simulink model "motion_detection"  (Simulink 7.3)
settings: Solver=ode45  StartTime=0.0  StopTime=15  RelTol=1e-3
undefined symbols (not defined in the file): Rec, SDTV, ttNCM
libraries: truetime x9, dspsigops x6, vipconversions x4, vipanalysis x4, vipgeotforms x4, dspobslib x4, dspsrcs4 x4, vipsnks x1
settings Model: Creator=Ayush Gupta  LastModifiedBy=Ayush Gupta
settings SimEventsCC: propDiagAttribOutput=1  propDiagFcnCallOutput=1  propDiagStatOutput=0

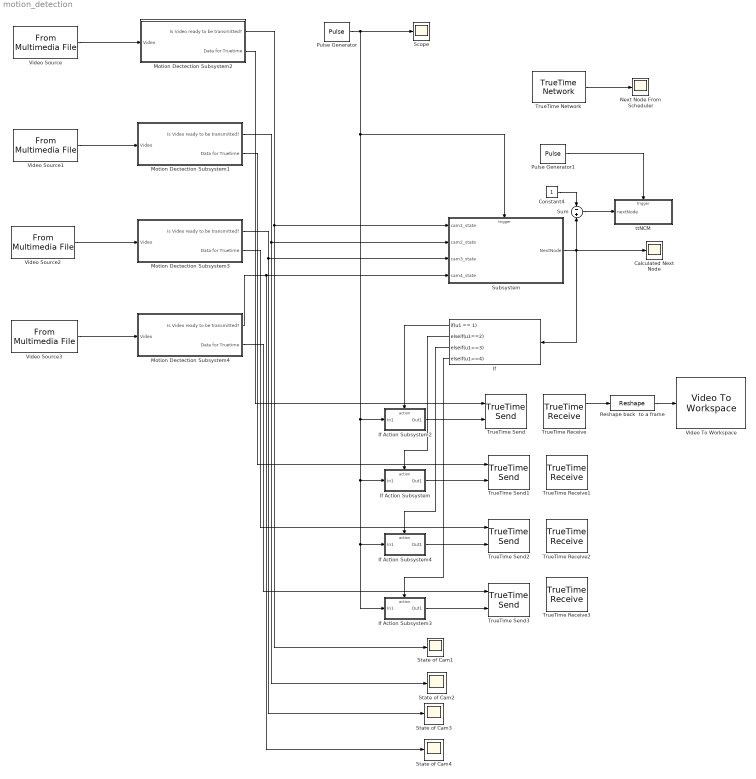
== system motion_detection ==
  Calculated Next Node : Scope
      settings: YMin=0  YMax=4
  Constant4 : Constant  OutDataType=fixdt(1, 16)  OutScaling=2^0
  If : If  IfExpression=u1 == 1  ElseIfExpressions=u1==2,u1==3,u1==4  ShowElse=off
  If Action Subsystem : Subsystem  TreatAsAtomicUnit=on
  If Action Subsystem2 : Subsystem  TreatAsAtomicUnit=on
  If Action Subsystem3 : Subsystem  TreatAsAtomicUnit=on
  If Action Subsystem4 : Subsystem  TreatAsAtomicUnit=on
  Motion Dectection Subsystem1 : Subsystem
  Motion Dectection Subsystem2 : Subsystem
  Motion Dectection Subsystem3 : Subsystem
  Motion Dectection Subsystem4 : Subsystem
  Next Node From Scheduler : Scope
      settings: YMin=1  YMax=4.5  SaveName=ScopeData5
  Pulse Generator : DiscretePulseGenerator  PulseType=Time based  Amplitude=1  Period=0.1  PulseWidth=10  PhaseDelay=0  SampleTime=1
  Pulse Generator1 : DiscretePulseGenerator  PulseType=Time based  Amplitude=1  Period=0.05  PulseWidth=10  PhaseDelay=0  SampleTime=1
  Reshape back  to a frame : Reshape  OutputDimensionality=Customize  OutputDimensions=[120,160,3]
  Scope : Scope
      settings: YMin=-1  YMax=1
  State of Cam{1..4} (4 alike) : Scope
      State of Cam1 settings: YMin=0  YMax=4  SaveName=ScopeData2
      State of Cam2 settings: YMin=0  YMax=4  SaveName=ScopeData3
      State of Cam3 settings: YMin=0  YMax=4  SaveName=ScopeData4
      State of Cam4 settings: YMin=0  YMax=4  SaveName=ScopeData6
  Subsystem : Subsystem
      settings: MinAlgLoopOccurrences=on
  Sum : Sum  Inputs=-+  OutDataType=sfix(16)  OutScaling=2^0  OutDataTypeStr=Inherit: Same as first input
  TrueTime Network : truetime/TrueTime Network  SystemSampleTime=-1  nwtype=NCM  nwnbr=1  nnodes=4  rate=10000  minsize=512  lossprob=0  seed=0  bandwidths=[0.5 0.5]  slotsize=512  schedule=[1 1 2]  memsize=80000  buftype=Common buffer  overflow=Retransmit  dynSchedule=0  miniSlotSize=0  NIT=0  QSortMode=FIFO  sync=0  irtSchedule=0  nrtLength=0  nodeGraph=0  scheduleoutput=on
  TrueTime Receive : truetime/TrueTime Receive  SystemSampleTime=-1  nwnbr=1  receiver=1  outdim=57600  triggeroutput=on  senderoutput=off  lengthoutput=off  priorityoutput=off  timestampoutput=off  signalpoweroutput=off  msgIDoutput=off
  TrueTime Receive1 : truetime/TrueTime Receive  SystemSampleTime=-1  nwnbr=1  receiver=2  outdim=57600  triggeroutput=on  senderoutput=off  lengthoutput=off  priorityoutput=off  timestampoutput=off  signalpoweroutput=off  msgIDoutput=off
  TrueTime Receive2 : truetime/TrueTime Receive  SystemSampleTime=-1  nwnbr=1  receiver=3  outdim=57600  triggeroutput=on  senderoutput=off  lengthoutput=off  priorityoutput=off  timestampoutput=off  signalpoweroutput=off  msgIDoutput=off
  TrueTime Receive3 : truetime/TrueTime Receive  SystemSampleTime=-1  nwnbr=1  receiver=4  outdim=57600  triggeroutput=on  senderoutput=off  lengthoutput=off  priorityoutput=off  timestampoutput=off  signalpoweroutput=off  msgIDoutput=off
  TrueTime Send : truetime/TrueTime Send  SystemSampleTime=-1  trigger=falling  nwnbr=1  sender=1  indim=57600  recsource=internal  receiver=1  lengthsource=internal  length=1000  priosource=internal  prio=1  msgIDsource=internal  msgID=0  dynamicSegment=dynamic
  TrueTime Send1 : truetime/TrueTime Send  SystemSampleTime=-1  trigger=falling  nwnbr=1  sender=2  indim=57600  recsource=internal  receiver=1  lengthsource=internal  length=1000  priosource=internal  prio=1  msgIDsource=internal  msgID=0  dynamicSegment=dynamic
  TrueTime Send2 : truetime/TrueTime Send  SystemSampleTime=-1  trigger=falling  nwnbr=1  sender=3  indim=57600  recsource=internal  receiver=1  lengthsource=internal  length=1000  priosource=internal  prio=1  msgIDsource=internal  msgID=0  dynamicSegment=dynamic
  TrueTime Send3 : truetime/TrueTime Send  SystemSampleTime=-1  trigger=falling  nwnbr=1  sender=4  indim=57600  recsource=internal  receiver=1  lengthsource=internal  length=1000  priosource=internal  prio=1  msgIDsource=internal  msgID=0  dynamicSegment=dynamic
  Video Source : dspsrcs4/From Multimedia File  DialogController=dspDDGCreate  DialogControllerArgs=DataTag8  inputFilename=C:\Users\Ayush Gupta\truetime\examples\NCM\VideoModel\InputVideo\vipmen.avi  loop=on  numPlays=inf  outputStreams=Video only  videoDataType=double  audioDataType=int16  inheritSampleTime=on  userDefinedSampleTime=1/30  noAudioOutput=off  isIntensityVideo=off  colorVideoFormat=One multidimensional signal  outputEOF=off  dataOrg=Column-major  audioFrameSize=1024
  Video Source1 : dspsrcs4/From Multimedia File  DialogController=dspDDGCreate  DialogControllerArgs=DataTag9  inputFilename=C:\Users\Ayush Gupta\truetime\examples\NCM\VideoModel\InputVideo\viptraffic.avi  loop=on  numPlays=inf  outputStreams=Video only  videoDataType=double  audioDataType=int16  inheritSampleTime=on  userDefinedSampleTime=1/30  noAudioOutput=off  isIntensityVideo=off  colorVideoFormat=One multidimensional signal  outputEOF=off  dataOrg=Column-major  audioFrameSize=1024
  Video Source2 : dspsrcs4/From Multimedia File  DialogController=dspDDGCreate  DialogControllerArgs=DataTag10  inputFilename=C:\Users\Ayush Gupta\truetime\examples\NCM\VideoModel\InputVideo\Surveillance1.wmv  loop=on  numPlays=inf  outputStreams=Video only  videoDataType=double  audioDataType=int16  inheritSampleTime=on  userDefinedSampleTime=1/30  noAudioOutput=off  isIntensityVideo=off  colorVideoFormat=One multidimensional signal  outputEOF=off  dataOrg=Column-major  audioFrameSize=1024
  Video Source3 : dspsrcs4/From Multimedia File  DialogController=dspDDGCreate  DialogControllerArgs=DataTag11  inputFilename=C:\Users\Ayush Gupta\truetime\examples\NCM\VideoModel\InputVideo\Surveillance2.wmv  loop=on  numPlays=inf  outputStreams=Video only  videoDataType=double  audioDataType=int16  inheritSampleTime=on  userDefinedSampleTime=1/30  noAudioOutput=off  isIntensityVideo=off  colorVideoFormat=One multidimensional signal  outputEOF=off  dataOrg=Column-major  audioFrameSize=1024
  Video To Workspace : vipsnks/Video To Workspace  DialogController=vipDDGCreate  DialogControllerArgs=DataTag12  VariableName=TestVideo  NumInputs=1  DataLimit=inf  DecimationFactor=1  LogFi=off  InPortLabels=R|G|B
  ttNCM : Subsystem  mask(ttNCM Wrapper){nNbr=1}
      mask prompts: nNbr "networkNbr"
      mask help: Specify the Network Number
  wires:
  Video Source/1 -> Motion Dectection Subsystem2/1(Video)
  Motion Dectection Subsystem2/1(Is Video ready to be transmitted?) -> Subsystem/1(cam1_state), State of Cam1/1
  Pulse Generator/1 -> Scope/1, Subsystem/Trigger, If Action Subsystem3/1(In1), If Action Subsystem4/1(In1), If Action Subsystem/1(In1), If Action Subsystem2/1(In1)
  Subsystem/1(NextNode) -> If/1, Calculated Next Node/1, Sum/2
  If Action Subsystem2/1(Out1) -> TrueTime Send/2
  If Action Subsystem/1(Out1) -> TrueTime Send1/2
  If Action Subsystem4/1(Out1) -> TrueTime Send2/2
  If Action Subsystem3/1(Out1) -> TrueTime Send3/2
  TrueTime Network/1 -> Next Node From Scheduler/1
  Constant4/1 -> Sum/1
  Sum/1 -> ttNCM/1(nextNode)
  Pulse Generator1/1 -> ttNCM/Trigger
  TrueTime Receive/1 -> Reshape back  to a frame/1
  Reshape back  to a frame/1 -> Video To Workspace/1
  Video Source3/1 -> Motion Dectection Subsystem4/1(Video)
  Video Source2/1 -> Motion Dectection Subsystem3/1(Video)
  Video Source1/1 -> Motion Dectection Subsystem1/1(Video)
  Motion Dectection Subsystem1/1(Is Video ready to be transmitted?) -> Subsystem/2(cam2_state), State of Cam2/1
  Motion Dectection Subsystem3/1(Is Video ready to be transmitted?) -> Subsystem/3(cam3_state), State of Cam3/1
  Motion Dectection Subsystem2/2(Data for Truetime) -> TrueTime Send/1
  Motion Dectection Subsystem4/1(Is Video ready to be transmitted?) -> Subsystem/4(cam4_state), State of Cam4/1
  If/1 -> If Action Subsystem2/Action
  If/2 -> If Action Subsystem/Action
  If/3 -> If Action Subsystem4/Action
  If/4 -> If Action Subsystem3/Action
  Motion Dectection Subsystem1/2(Data for Truetime) -> TrueTime Send1/1
  Motion Dectection Subsystem3/2(Data for Truetime) -> TrueTime Send2/1
  Motion Dectection Subsystem4/2(Data for Truetime) -> TrueTime Send3/1

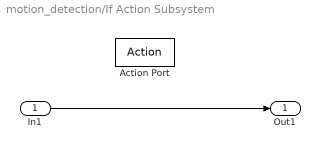
== system motion_detection/If Action Subsystem ==
  In1 : Inport  OutDataType=fixdt(1, 16)  OutScaling=2^0
  Action Port : ActionPort  ActionType=elseif
  Out1 : Outport  OutDataType=fixdt(1, 16)  OutScaling=2^0
  wires:
  In1/1 -> Out1/1

== system motion_detection/If Action Subsystem2 ==
  In1 : Inport  OutDataType=fixdt(1, 16)  OutScaling=2^0
  Action Port : ActionPort  ActionType=then
  Out1 : Outport  OutDataType=fixdt(1, 16)  OutScaling=2^0
  wires:
  In1/1 -> Out1/1

== system motion_detection/If Action Subsystem3 ==
  In1 : Inport  OutDataType=fixdt(1, 16)  OutScaling=2^0
  Action Port : ActionPort  ActionType=elseif
  Out1 : Outport  OutDataType=fixdt(1, 16)  OutScaling=2^0
  wires:
  In1/1 -> Out1/1

== system motion_detection/If Action Subsystem4 ==
  In1 : Inport  OutDataType=fixdt(1, 16)  OutScaling=2^0
  Action Port : ActionPort  ActionType=elseif
  Out1 : Outport  OutDataType=fixdt(1, 16)  OutScaling=2^0
  wires:
  In1/1 -> Out1/1

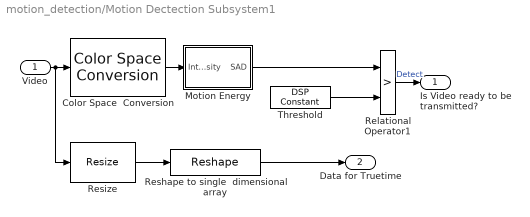
== system motion_detection/Motion Dectection Subsystem1 ==
  Video : Inport
  Color Space  Conversion : vipconversions/Color Space  Conversion  conversion=Obsolete  conversionActive=R'G'B' to intensity  wp_str=D65  rec=Rec. 601 (SDTV)  sys=1125/60/2:1  imagePorts=One multidimensional signal
  Motion Energy : Subsystem
  Relational Operator1 : RelationalOperator  Operator=>  LogicOutDataTypeMode=boolean  OutDataTypeStr=boolean  InputSameDT=on
  Reshape to single  dimensional array : Reshape
  Resize : vipgeotforms/Resize  DialogController=vipDDGCreate  DialogControllerArgs=DataTag1  specify=Number of output rows and columns  rfactor=[200 150]  outCols=25  outRows=25  outRowsCols=[120 160]  interp_method=Bilinear  antialias=on  useROI=off  roiFlag=off  prodOutputMode=Binary point scaling  prodOutputWordLength=32  prodOutputFracLength=10  roundingMode=Nearest  overflowMode=on
  Threshold : dspobslib/DSP Constant  SystemSampleTime=-1  Value=1e5/(255)  SampleMode=Discrete  discreteOutput=Sample-based  continuousOutput=Sample-based  sampTime=inf  framePeriod=inf  dataType=Inherit via back propagation  isSigned=on  wordLen=16  udDataType=sfix(16)  fracBitsMode=Best precision  numFracBits=15  InterpretAs1D=off  Ts=inf  FramebasedOutput=off
      settings: additionalParams=on
  Is Video ready to be transmitted? : Outport
  Data for Truetime : Outport  Port=2
  wires:
  Motion Energy/1(SAD) -> Relational Operator1/1
  Threshold/1 -> Relational Operator1/2
  Video/1 -> Color Space  Conversion/1, Resize/1
  Relational Operator1/1 -> Is Video ready to be transmitted?/1  "Detect"
  Color Space  Conversion/1 -> Motion Energy/1(Intensity)
  Reshape to single  dimensional array/1 -> Data for Truetime/1
  Resize/1 -> Reshape to single  dimensional array/1

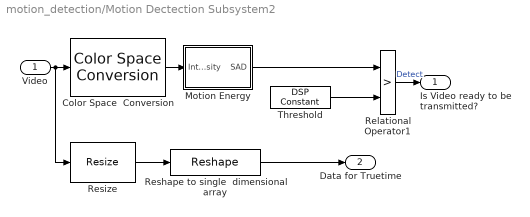
== system motion_detection/Motion Dectection Subsystem2 ==
  Video : Inport
  Color Space  Conversion : vipconversions/Color Space  Conversion  conversion=Obsolete  conversionActive=R'G'B' to intensity  wp_str=D65  rec=Rec. 601 (SDTV)  sys=1125/60/2:1  imagePorts=One multidimensional signal
  Motion Energy : Subsystem
  Relational Operator1 : RelationalOperator  Operator=>  LogicOutDataTypeMode=boolean  OutDataTypeStr=boolean  InputSameDT=on
  Reshape to single  dimensional array : Reshape
  Resize : vipgeotforms/Resize  DialogController=vipDDGCreate  DialogControllerArgs=DataTag3  specify=Number of output rows and columns  rfactor=[200 150]  outCols=25  outRows=25  outRowsCols=[120 160]  interp_method=Bilinear  antialias=on  useROI=off  roiFlag=off  prodOutputMode=Binary point scaling  prodOutputWordLength=32  prodOutputFracLength=10  roundingMode=Nearest  overflowMode=on
  Threshold : dspobslib/DSP Constant  SystemSampleTime=-1  Value=1e5/(255)  SampleMode=Discrete  discreteOutput=Sample-based  continuousOutput=Sample-based  sampTime=inf  framePeriod=inf  dataType=Inherit via back propagation  isSigned=on  wordLen=16  udDataType=sfix(16)  fracBitsMode=Best precision  numFracBits=15  InterpretAs1D=off  Ts=inf  FramebasedOutput=off
      settings: additionalParams=on
  Is Video ready to be transmitted? : Outport
  Data for Truetime : Outport  Port=2
  wires:
  Motion Energy/1(SAD) -> Relational Operator1/1
  Threshold/1 -> Relational Operator1/2
  Video/1 -> Color Space  Conversion/1, Resize/1
  Relational Operator1/1 -> Is Video ready to be transmitted?/1  "Detect"
  Color Space  Conversion/1 -> Motion Energy/1(Intensity)
  Reshape to single  dimensional array/1 -> Data for Truetime/1
  Resize/1 -> Reshape to single  dimensional array/1

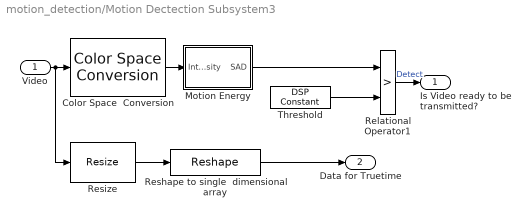
== system motion_detection/Motion Dectection Subsystem3 ==
  Video : Inport
  Color Space  Conversion : vipconversions/Color Space  Conversion  conversion=Obsolete  conversionActive=R'G'B' to intensity  wp_str=D65  rec=Rec. 601 (SDTV)  sys=1125/60/2:1  imagePorts=One multidimensional signal
  Motion Energy : Subsystem
  Relational Operator1 : RelationalOperator  Operator=>  LogicOutDataTypeMode=boolean  OutDataTypeStr=boolean  InputSameDT=on
  Reshape to single  dimensional array : Reshape
  Resize : vipgeotforms/Resize  DialogController=vipDDGCreate  DialogControllerArgs=DataTag5  specify=Number of output rows and columns  rfactor=[200 150]  outCols=25  outRows=25  outRowsCols=[120 160]  interp_method=Bilinear  antialias=on  useROI=off  roiFlag=off  prodOutputMode=Binary point scaling  prodOutputWordLength=32  prodOutputFracLength=10  roundingMode=Nearest  overflowMode=on
  Threshold : dspobslib/DSP Constant  SystemSampleTime=-1  Value=1e5/(255)  SampleMode=Discrete  discreteOutput=Sample-based  continuousOutput=Sample-based  sampTime=inf  framePeriod=inf  dataType=Inherit via back propagation  isSigned=on  wordLen=16  udDataType=sfix(16)  fracBitsMode=Best precision  numFracBits=15  InterpretAs1D=off  Ts=inf  FramebasedOutput=off
      settings: additionalParams=on
  Is Video ready to be transmitted? : Outport
  Data for Truetime : Outport  Port=2
  wires:
  Motion Energy/1(SAD) -> Relational Operator1/1
  Threshold/1 -> Relational Operator1/2
  Video/1 -> Color Space  Conversion/1, Resize/1
  Relational Operator1/1 -> Is Video ready to be transmitted?/1  "Detect"
  Color Space  Conversion/1 -> Motion Energy/1(Intensity)
  Reshape to single  dimensional array/1 -> Data for Truetime/1
  Resize/1 -> Reshape to single  dimensional array/1

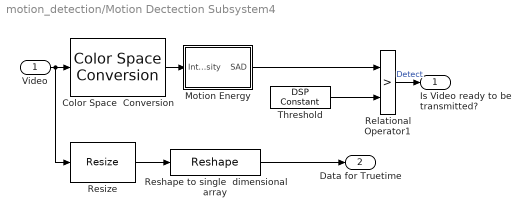
== system motion_detection/Motion Dectection Subsystem4 ==
  Video : Inport
  Color Space  Conversion : vipconversions/Color Space  Conversion  conversion=Obsolete  conversionActive=R'G'B' to intensity  wp_str=D65  rec=Rec. 601 (SDTV)  sys=1125/60/2:1  imagePorts=One multidimensional signal
  Motion Energy : Subsystem
  Relational Operator1 : RelationalOperator  Operator=>  LogicOutDataTypeMode=boolean  OutDataTypeStr=boolean  InputSameDT=on
  Reshape to single  dimensional array : Reshape
  Resize : vipgeotforms/Resize  DialogController=vipDDGCreate  DialogControllerArgs=DataTag7  specify=Number of output rows and columns  rfactor=[200 150]  outCols=25  outRows=25  outRowsCols=[120 160]  interp_method=Bilinear  antialias=on  useROI=off  roiFlag=off  prodOutputMode=Binary point scaling  prodOutputWordLength=32  prodOutputFracLength=10  roundingMode=Nearest  overflowMode=on
  Threshold : dspobslib/DSP Constant  SystemSampleTime=-1  Value=1e5/(255)  SampleMode=Discrete  discreteOutput=Sample-based  continuousOutput=Sample-based  sampTime=inf  framePeriod=inf  dataType=Inherit via back propagation  isSigned=on  wordLen=16  udDataType=sfix(16)  fracBitsMode=Best precision  numFracBits=15  InterpretAs1D=off  Ts=inf  FramebasedOutput=off
      settings: additionalParams=on
  Is Video ready to be transmitted? : Outport
  Data for Truetime : Outport  Port=2
  wires:
  Motion Energy/1(SAD) -> Relational Operator1/1
  Threshold/1 -> Relational Operator1/2
  Video/1 -> Color Space  Conversion/1, Resize/1
  Relational Operator1/1 -> Is Video ready to be transmitted?/1  "Detect"
  Color Space  Conversion/1 -> Motion Energy/1(Intensity)
  Reshape to single  dimensional array/1 -> Data for Truetime/1
  Resize/1 -> Reshape to single  dimensional array/1

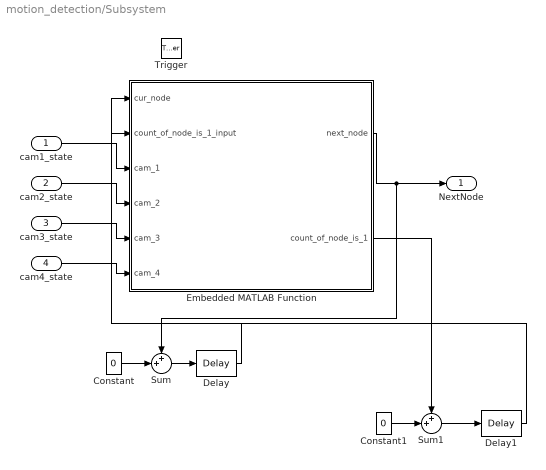
== system motion_detection/Subsystem ==
  cam1_state : Inport  OutDataType=fixdt(1, 16)  OutScaling=2^0
  cam2_state : Inport  Port=2  OutDataType=fixdt(1, 16)  OutScaling=2^0
  cam3_state : Inport  Port=3  OutDataType=fixdt(1, 16)  OutScaling=2^0
  cam4_state : Inport  Port=4  OutDataType=fixdt(1, 16)  OutScaling=2^0
  Trigger : TriggerPort  TriggerType=falling
  Constant : Constant  Value=0  OutDataTypeMode=int32  OutDataType=sfix(16)  OutScaling=2^0  OutDataTypeStr=int32
  Constant1 : Constant  Value=0  OutDataTypeMode=int32  OutDataType=sfix(16)  OutScaling=2^0  OutDataTypeStr=int32
  Delay : dspsigops/Delay  dly_unit=Samples  delay=1  ic_detail=off  dif_ic_for_ch=off  dif_ic_for_dly=off  ic=0  reset_popup=None
  Delay1 : dspsigops/Delay  dly_unit=Samples  delay=1  ic_detail=off  dif_ic_for_ch=off  dif_ic_for_dly=off  ic=0  reset_popup=None
  Embedded MATLAB Function : Stateflow chart
  Sum : Sum  Inputs=++|  OutDataType=sfix(16)  OutScaling=2^0  OutDataTypeStr=Inherit: Same as first input
  Sum1 : Sum  Inputs=++|  OutDataType=sfix(16)  OutScaling=2^0  OutDataTypeStr=Inherit: Same as first input
  NextNode : Outport  OutDataType=fixdt(1, 16)  OutScaling=2^0
  wires:
  cam1_state/1 -> Embedded MATLAB Function/3(cam_1)
  cam2_state/1 -> Embedded MATLAB Function/4(cam_2)
  cam3_state/1 -> Embedded MATLAB Function/5(cam_3)
  cam4_state/1 -> Embedded MATLAB Function/6(cam_4)
  Embedded MATLAB Function/1(next_node) -> NextNode/1, Sum/1
  Constant/1 -> Sum/2
  Constant1/1 -> Sum1/2
  Sum/1 -> Delay/1
  Embedded MATLAB Function/2(count_of_node_is_1) -> Sum1/1
  Sum1/1 -> Delay1/1
  Delay/1 -> Embedded MATLAB Function/1(cur_node)
  Delay1/1 -> Embedded MATLAB Function/2(count_of_node_is_1_input)

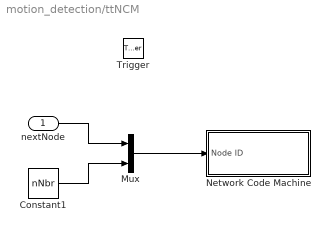
== system motion_detection/ttNCM ==
  nextNode : Inport  OutDataType=fixdt(1, 16)  OutScaling=2^0
  Trigger : TriggerPort  TriggerType=either
  Constant1 : Constant  Value=nNbr  OutDataType=fixdt(1, 16)  OutScaling=2^0
  Mux : Mux  Inputs=2
  Network Code Machine : Subsystem  AncestorBlock=NCM/Network Code Machine  TreatAsAtomicUnit=on
  wires:
  nextNode/1 -> Mux/1
  Constant1/1 -> Mux/2
  Mux/1 -> Network Code Machine/1(Node ID)

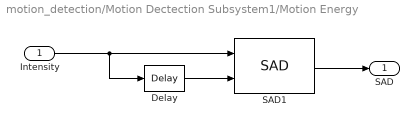
== system motion_detection/Motion Dectection Subsystem1/Motion Energy ==
  Intensity : Inport  OutDataType=sfix(16)  OutScaling=2^0
  Delay : dspsigops/Delay  dly_unit=Samples  delay=1  ic_detail=off  dif_ic_for_ch=off  dif_ic_for_dly=off  ic=0  reset_popup=None
  SAD1 : vipanalysis/SAD  DialogController=vipDDGCreate  DialogControllerArgs=DataTag0  output=SAD values  method=Exhaustive  roi=off  invalidROI=Ignore  nearbyPel=off  nearbySize=3  roundingMode=Floor  overflowMode=off
  SAD : Outport  OutDataType=sfix(16)  OutScaling=2^0
  wires:
  Intensity/1 -> SAD1/1, Delay/1
  Delay/1 -> SAD1/2
  SAD1/1 -> SAD/1

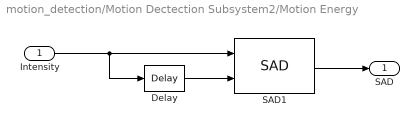
== system motion_detection/Motion Dectection Subsystem2/Motion Energy ==
  Intensity : Inport  OutDataType=sfix(16)  OutScaling=2^0
  Delay : dspsigops/Delay  dly_unit=Samples  delay=1  ic_detail=off  dif_ic_for_ch=off  dif_ic_for_dly=off  ic=0  reset_popup=None
  SAD1 : vipanalysis/SAD  DialogController=vipDDGCreate  DialogControllerArgs=DataTag2  output=SAD values  method=Exhaustive  roi=off  invalidROI=Ignore  nearbyPel=off  nearbySize=3  roundingMode=Floor  overflowMode=off
  SAD : Outport  OutDataType=sfix(16)  OutScaling=2^0
  wires:
  Intensity/1 -> SAD1/1, Delay/1
  Delay/1 -> SAD1/2
  SAD1/1 -> SAD/1

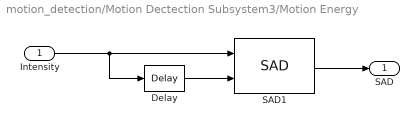
== system motion_detection/Motion Dectection Subsystem3/Motion Energy ==
  Intensity : Inport  OutDataType=sfix(16)  OutScaling=2^0
  Delay : dspsigops/Delay  dly_unit=Samples  delay=1  ic_detail=off  dif_ic_for_ch=off  dif_ic_for_dly=off  ic=0  reset_popup=None
  SAD1 : vipanalysis/SAD  DialogController=vipDDGCreate  DialogControllerArgs=DataTag4  output=SAD values  method=Exhaustive  roi=off  invalidROI=Ignore  nearbyPel=off  nearbySize=3  roundingMode=Floor  overflowMode=off
  SAD : Outport  OutDataType=sfix(16)  OutScaling=2^0
  wires:
  Intensity/1 -> SAD1/1, Delay/1
  Delay/1 -> SAD1/2
  SAD1/1 -> SAD/1

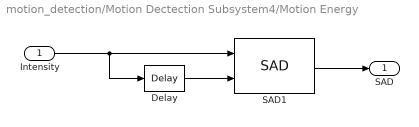
== system motion_detection/Motion Dectection Subsystem4/Motion Energy ==
  Intensity : Inport  OutDataType=sfix(16)  OutScaling=2^0
  Delay : dspsigops/Delay  dly_unit=Samples  delay=1  ic_detail=off  dif_ic_for_ch=off  dif_ic_for_dly=off  ic=0  reset_popup=None
  SAD1 : vipanalysis/SAD  DialogController=vipDDGCreate  DialogControllerArgs=DataTag6  output=SAD values  method=Exhaustive  roi=off  invalidROI=Ignore  nearbyPel=off  nearbySize=3  roundingMode=Floor  overflowMode=off
  SAD : Outport  OutDataType=sfix(16)  OutScaling=2^0
  wires:
  Intensity/1 -> SAD1/1, Delay/1
  Delay/1 -> SAD1/2
  SAD1/1 -> SAD/1

== system motion_detection/ttNCM/Network Code Machine ==
  Node ID : Inport
  MATLAB Fcn : MATLABFcn  MATLABFcn=ttNCM(u(1),u(2))  OutputDimensions=0
  wires:
  Node ID/1 -> MATLAB Fcn/1

== matlab function Subsystem/Embedded MATLAB Function ==
  data: cur_node input double; count_of_node_is_1_input input double; next_node output double; cam_1 input double; cam_2 input double; cam_3 input double; cam_4 input double; count_of_node_is_1 output double
function [ next_node , count_of_node_is_1] = CalculateNextVideo(cur_node, count_of_node_is_1_input , cam_1, cam_2 , cam_3, cam_4)
MAX_NODES = 4;
MAX_FRAMES = 5;
camera_cond = [ cam_1, cam_2, cam_3, cam_4];   
% Initial Condition 
if ( cur_node < 1 || cur_node > MAX_NODES  )
    next_node = 1;
    count_of_node_is_1 = MAX_FRAMES;
    return;
end

% Rounding to ensure we get integers
cur_node_counter = round(cur_node);

% Transmit atleast 5 more frames from the camera after the object has been removed
if ( count_of_node_is_1_input < MAX_FRAMES )
    next_node = cur_node_counter;
    count_of_node_is_1 = count_of_node_is_1_input + 1
    return;
else
    count_of_node_is_1 = MAX_FRAMES;
end

% Checking which cameras have an object in front of them
% The algorithm follows, if the current node is ready to transmit, then
% transmit, else transmit other nodes
for counter = 1:MAX_NODES
    if ( cur_node_counter == MAX_NODES + 1 )
        cur_node_counter = 1;
    end
    
    if ( camera_cond(counter) == 1 ) 
        next_node = counter;
        count_of_node_is_1 = 0;  % This outputs that the current node now set is choosen because it had an object
        return;
    end
    
    cur_node_counter = cur_node_counter+1;
end

% If there is no need with object in front of them, then transmit next node.
 if ( cur_node_counter == MAX_NODES )
        cur_node_counter = 0;
 end
    
next_node = cur_node_counter + 1;
return
